simulink model "SIG_A_construction_updated"  (R2014b)
settings: Solver=ode45  StartTime=0.0  StopTime=10.0  RelTol=1e-3
libraries: dspindex x3, commofdm x2, commcnvcod2 x1, commdigbbndpm3 x1
settings Model: Creator=Yuan  LastModifiedBy=Admin
settings DataIOCC: SaveFormat=Structure

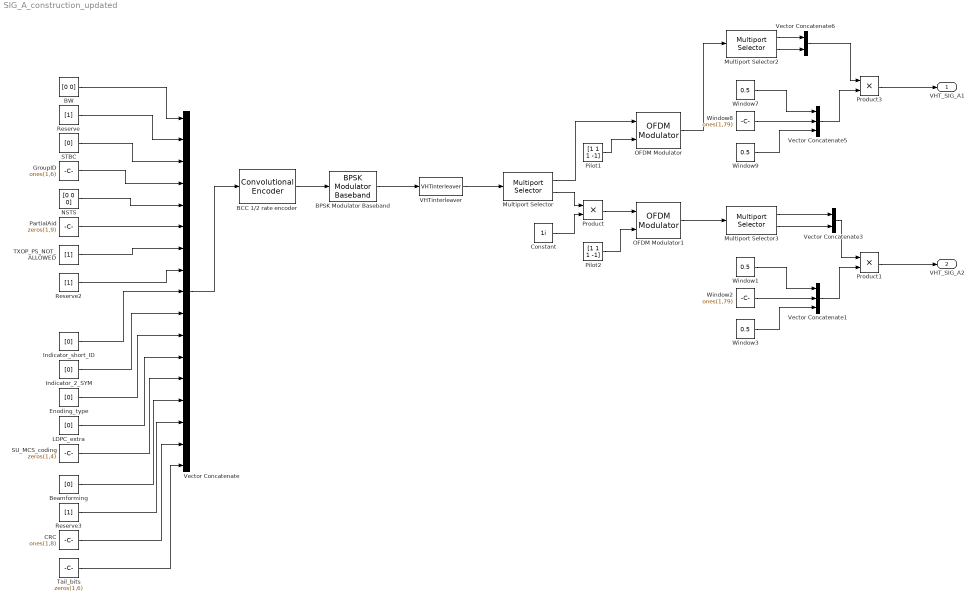
== system SIG_A_construction_updated ==
  BCC 1/2 rate encoder : commcnvcod2/Convolutional Encoder  trellis=poly2trellis(7, [133 171])  opMode=Continuous  DelayedResetAction=off  hasIniStPort=off  hasFinStPort=off  usePuncVector=on  punctureVector=[1]  reset=Unused parameter value
  BPSK Modulator Baseband : commdigbbndpm3/BPSK Modulator Baseband  Ph=pi  outDtype=Inherit via back propagation  outWordLen=16  outUDDataType=sfix(16)  outFracLenMode=Best precision  outFracLen=15
  BW : Constant  Value=[0 0]  SampleTime=1
  Beamforming : Constant  Value=[0]  SampleTime=1
  CRC : Constant  Value=ones(1,8)  SampleTime=1
  Constant : Constant  Value=1i  SampleTime=1
  Enoding_type : Constant  Value=[0]  SampleTime=1
  GroupID : Constant  Value=ones(1,6)  SampleTime=1
  Indicator_2_SYM : Constant  Value=[0]  SampleTime=1
  Indicator_short_ID : Constant  Value=[0]  SampleTime=1
  LDPC_extra : Constant  Value=[0]  SampleTime=1
  Multiport Selector : dspindex/Multiport Selector  rowsOrCols=Rows  idxCellArray={[1:48], [49:96]}  idxErrMode=Clip Index
  Multiport Selector2 : dspindex/Multiport Selector  rowsOrCols=Rows  idxCellArray={ [1:80],17 }  idxErrMode=Clip Index
  Multiport Selector3 : dspindex/Multiport Selector  rowsOrCols=Rows  idxCellArray={ [1:80],17 }  idxErrMode=Clip Index
  NSTS : Constant  Value=[0 0 0]  SampleTime=1
  OFDM Modulator : commofdm/OFDM Modulator  SimulateUsing=Interpreted execution  FFTLength=64  NumGuardBandCarriers=[6; 5]  InsertDCNull=on  PilotInputPort=on  PilotCarrierIndices=[12; 26; 40; 54]  CyclicPrefixLength=16  Windowing=off  WindowLength=1  NumSymbols=1  NumTransmitAntennas=1
  OFDM Modulator1 : commofdm/OFDM Modulator  SimulateUsing=Interpreted execution  FFTLength=64  NumGuardBandCarriers=[6; 5]  InsertDCNull=on  PilotInputPort=on  PilotCarrierIndices=[12; 26; 40; 54]  CyclicPrefixLength=16  Windowing=off  WindowLength=1  NumSymbols=1  NumTransmitAntennas=1
  PartialAid : Constant  Value=zeros(1,9)  SampleTime=1
  Pilot1 : Constant  Value=[1 1 1 -1]  SampleTime=1
  Pilot2 : Constant  Value=[1 1 1 -1]  SampleTime=1
  Product : Product  SampleTime=1
  Product1 : Product  SampleTime=1
  Product3 : Product  SampleTime=1
  Reserve : Constant  Value=[1]  SampleTime=1
  Reserve2 : Constant  Value=[1]  SampleTime=1
  Reserve3 : Constant  Value=[1]  SampleTime=1
  STBC : Constant  Value=[0]  SampleTime=1
  SU_MCS_coding : Constant  Value=zeros(1,4)  SampleTime=1
  TXOP_PS_NOT_ALLOWED : Constant  Value=[1]  SampleTime=1
  Tail_bits : Constant  Value=zeros(1,6)  SampleTime=1
  VHTinterleaver : MATLABFcn  MATLABFcn=VHTinterleaver  OutputSignalType=complex
  Vector Concatenate : Concatenate  NumInputs=17
  Vector Concatenate1 : Concatenate  NumInputs=3
  Vector Concatenate3 : Concatenate
  Vector Concatenate5 : Concatenate  NumInputs=3
  Vector Concatenate6 : Concatenate
  Window{1,3,7,9} (4 alike) : Constant  Value=0.5  SampleTime=1
  Window2 : Constant  Value=ones(1,79)  SampleTime=1
  Window8 : Constant  Value=ones(1,79)  SampleTime=1
  VHT_SIG_A1 : Outport
  VHT_SIG_A2 : Outport  Port=2
  wires:
  BW/1 -> Vector Concatenate/1
  Reserve/1 -> Vector Concatenate/2
  STBC/1 -> Vector Concatenate/3
  GroupID/1 -> Vector Concatenate/4
  NSTS/1 -> Vector Concatenate/5
  PartialAid/1 -> Vector Concatenate/6
  TXOP_PS_NOT_ALLOWED/1 -> Vector Concatenate/7
  Reserve2/1 -> Vector Concatenate/8
  Vector Concatenate/1 -> BCC 1/2 rate encoder/1
  BPSK Modulator Baseband/1 -> VHTinterleaver/1
  BCC 1/2 rate encoder/1 -> BPSK Modulator Baseband/1
  Indicator_short_ID/1 -> Vector Concatenate/9
  Indicator_2_SYM/1 -> Vector Concatenate/10
  Enoding_type/1 -> Vector Concatenate/11
  LDPC_extra/1 -> Vector Concatenate/12
  SU_MCS_coding/1 -> Vector Concatenate/13
  Beamforming/1 -> Vector Concatenate/14
  Reserve3/1 -> Vector Concatenate/15
  CRC/1 -> Vector Concatenate/16
  Tail_bits/1 -> Vector Concatenate/17
  VHTinterleaver/1 -> Multiport Selector/1
  Multiport Selector/1 -> OFDM Modulator/1
  Pilot1/1 -> OFDM Modulator/2
  Multiport Selector/2 -> Product/1
  Constant/1 -> Product/2
  Product/1 -> OFDM Modulator1/1
  Pilot2/1 -> OFDM Modulator1/2
  OFDM Modulator1/1 -> Multiport Selector3/1
  Multiport Selector3/2 -> Vector Concatenate3/2
  Multiport Selector3/1 -> Vector Concatenate3/1
  Vector Concatenate3/1 -> Product1/1
  Window1/1 -> Vector Concatenate1/1
  Window2/1 -> Vector Concatenate1/2
  Window3/1 -> Vector Concatenate1/3
  Vector Concatenate1/1 -> Product1/2
  Multiport Selector2/2 -> Vector Concatenate6/2
  Multiport Selector2/1 -> Vector Concatenate6/1
  Vector Concatenate6/1 -> Product3/1
  Window7/1 -> Vector Concatenate5/1
  Window8/1 -> Vector Concatenate5/2
  Window9/1 -> Vector Concatenate5/3
  Vector Concatenate5/1 -> Product3/2
  OFDM Modulator/1 -> Multiport Selector2/1
  Product3/1 -> VHT_SIG_A1/1
  Product1/1 -> VHT_SIG_A2/1
